simulink model "test_viconFilter"  (Simulink 7.7)
settings: Solver=ode45  StartTime=0.0  StopTime=30  RelTol=1e-3
settings Model: Creator=Zhao Weihua  LastModifiedBy=Zhao Weihua

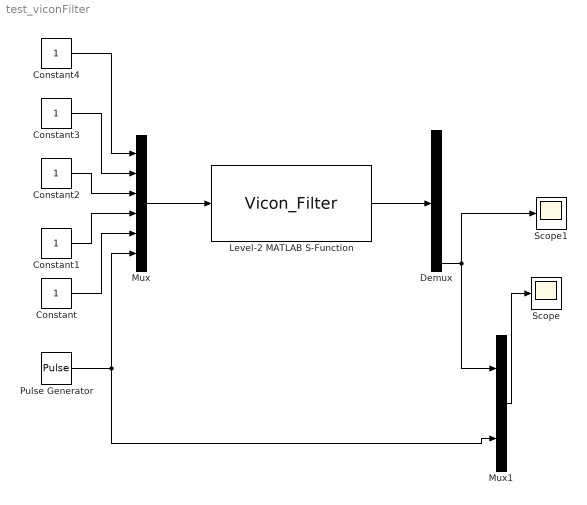
== system test_viconFilter ==
  Constant{,1..4} (5 alike) : Constant
  Demux : Demux  Outputs=6
  Level-2 MATLAB S-Function : M-S-Function  FunctionName=Vicon_Filter
  Mux : Mux  Inputs=6
  Mux1 : Mux  Inputs=2
  Pulse Generator : DiscretePulseGenerator  PulseType=Time based  Period=10  PulseWidth=0.1
  Scope : Scope
  Scope1 : Scope
  wires:
  Constant4/1 -> Mux/1
  Constant3/1 -> Mux/2
  Constant2/1 -> Mux/3
  Constant1/1 -> Mux/4
  Constant/1 -> Mux/5
  Pulse Generator/1 -> Mux/6, Mux1/2
  Mux/1 -> Level-2 MATLAB S-Function/1
  Level-2 MATLAB S-Function/1 -> Demux/1
  Demux/6 -> Mux1/1, Scope1/1
  Mux1/1 -> Scope/1
